simulink model "modelo_2_grados"  (R2021a)
settings: Solver=VariableStepAuto  StartTime=0.0  StopTime=10.0  RelTol=1e-3
values from neighbouring files (symbols this model uses):
  C = tf(K,1)    [ControlP.m]    (also in ControlPID.m = C_pid; DeadBeat.m = Fa)
  Cd = c2d(C,ts,'zoh')    [ControlP.m]    (also in ControlPID.m = Cd_pid; DeadBeat.m = minreal(F/(Pd-F*Pd)))
  Cr = C    [ControlP.m]    (also in ControlPID.m = Cr_pid; DeadBeat.m)
  Crd = Cd    [ControlP.m]    (also in ControlPID.m = Crd_pid; DeadBeat.m)
  Fa = tf(1,1)    [ControlP.m]    (also in ControlPID.m; DeadBeat.m)
  P = Km/(Tm*s+1)/(Tf*s+1)    [ControlP.m]    (also in ControlPID.m; DeadBeat.m; DesignP.m; todoModeloPrep.m = 50/((s+5)*(s+2)))
  Pd = c2d(P,ts)    [ControlP.m]    (also in ControlPID.m; DeadBeat.m = c2d(P, Ts, 'zoh'); DesignP.m = -P; todoModeloPrep.m)
  ret = 1    [ControlP.m]    (also in ControlPID.m = 0; DeadBeat.m = 0)
  Ts = ts    (= 0.1)    [ControlP.m]    (also in ControlPID.m = 0.03; DeadBeat.m = 0.105)
settings Model: Creator=ferna  LastModifiedBy=quint

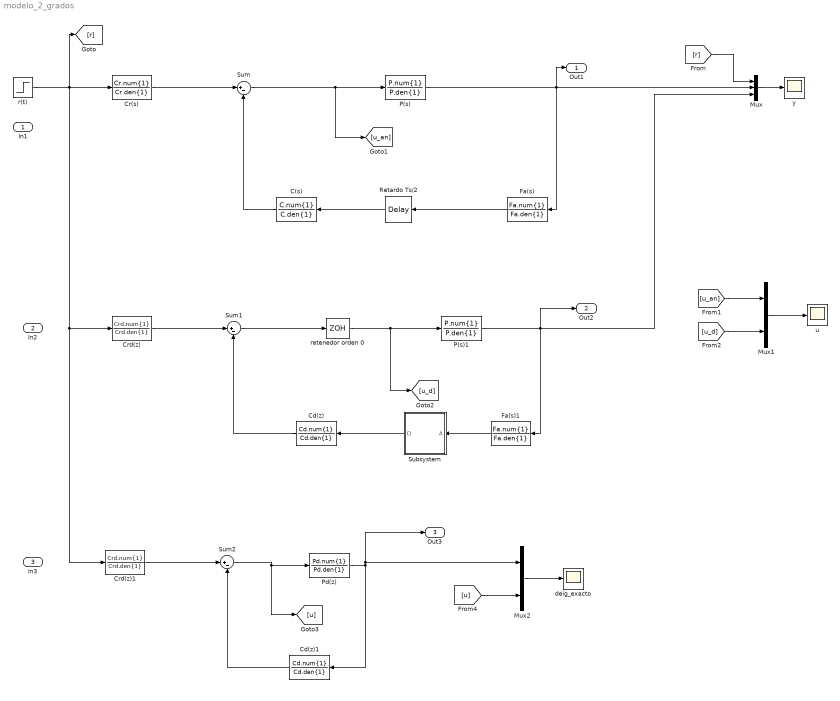
== system modelo_2_grados ==
  In1 : Inport
  In2 : Inport  Port=2
  In3 : Inport  Port=3
  C(s) : TransferFcn  Numerator=C.num{1}  Denominator=C.den{1}
  Cd(z) : DiscreteTransferFcn  Numerator=Cd.num{1}  Denominator=Cd.den{1}  SampleTime=Ts
  Cd(z)1 : DiscreteTransferFcn  Numerator=Cd.num{1}  Denominator=Cd.den{1}  SampleTime=Ts
  Cr(s) : TransferFcn  Numerator=Cr.num{1}  Denominator=Cr.den{1}
  Crd(z) : DiscreteTransferFcn  Numerator=Crd.num{1}  Denominator=Crd.den{1}  SampleTime=Ts
  Crd(z)1 : DiscreteTransferFcn  Numerator=Crd.num{1}  Denominator=Crd.den{1}  SampleTime=Ts
  Fa(s) : TransferFcn  Numerator=Fa.num{1}  Denominator=Fa.den{1}
  Fa(s)1 : TransferFcn  Numerator=Fa.num{1}  Denominator=Fa.den{1}
  Mux : Mux  Inputs=3
  Mux1 : Mux  Inputs=2
  Mux2 : Mux  Inputs=2
  P(s) : TransferFcn  Numerator=P.num{1}  Denominator=P.den{1}
  P(s)1 : TransferFcn  Numerator=P.num{1}  Denominator=P.den{1}
  Pd(z) : DiscreteTransferFcn  Numerator=Pd.num{1}  Denominator=Pd.den{1}  SampleTime=Ts
  Retardo Ts/2 : TransportDelay  DelayTime=ret*Ts/2
  Subsystem : Subsystem
  Sum : Sum  Inputs=|+-
  Sum1 : Sum  Inputs=|+-
  Sum2 : Sum  Inputs=|+-
  deig_exacto : Scope
  r(t) : Step  Time=0  SampleTime=0
  retenedor orden 0 : ZeroOrderHold  SampleTime=-1
  u : Scope
  y : Scope
  Out1 : Outport
  Out2 : Outport  Port=2
  Out3 : Outport  Port=3
  wires:
  Cr(s)/1 -> Sum/1
  C(s)/1 -> Sum/2
  Retardo Ts/2/1 -> C(s)/1
  Fa(s)/1 -> Retardo Ts/2/1
  P(s)/1 -> Out1/1, Fa(s)/1, Mux/2
  Sum/1 -> [u_an], P(s)/1
  Crd(z)/1 -> Sum1/1
  P(s)1/1 -> Out2/1, Mux/3, Fa(s)1/1
  Cd(z)/1 -> Sum1/2
  Sum1/1 -> retenedor orden 0/1
  retenedor orden 0/1 -> [u_d], P(s)1/1
  Subsystem/1(D) -> Cd(z)/1
  Fa(s)1/1 -> Subsystem/1(A)
  Crd(z)1/1 -> Sum2/1
  Cd(z)1/1 -> Sum2/2
  Sum2/1 -> [u], Pd(z)/1
  Pd(z)/1 -> Mux2/1, Out3/1, Cd(z)1/1
  [r] -> Mux/1
  Mux/1 -> y/1
  Mux1/1 -> u/1
  [u_d] -> Mux1/2
  [u_an] -> Mux1/1
  r(t)/1 -> [r], Crd(z)1/1, Crd(z)/1, Cr(s)/1
  Mux2/1 -> deig_exacto/1
  [u] -> Mux2/2

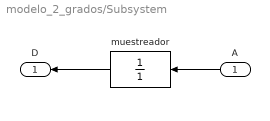
== system modelo_2_grados/Subsystem ==
  A : Inport
  muestreador : DiscreteTransferFcn  Denominator=[1]  SampleTime=Ts
  D : Outport
  wires:
  muestreador/1 -> D/1
  A/1 -> muestreador/1
